simulink model "deltino"  (R2021b)
settings: Solver=VariableStepAuto  StartTime=0.0  StopTime=inf  FixedStep=0.0001  RelTol=1e-3
values from neighbouring files (symbols this model uses):
  alpha1 = 0    [compute_deltino_dyn_parallel.m]
  alpha2 = 2/3*pi    (= 2.09439510239)    [compute_deltino_dyn_parallel.m]
  alpha3 = 4/3*pi    (= 4.18879020479)    [compute_deltino_dyn_parallel.m]
  H = 0.05    [main.m]
  J_T = [J_1', J_2', J_3', J_4']    [main.m]
  K_d = 10    [main.m]
  K_el = 10000    [main.m]
  K_i = 1    [main.m]
  K_p = 200    [main.m]
  K_v = 10    [main.m]
  mu = 0.8    [main.m]
  ni_0 = zeros(18,1)    [main.m]
  offset1 = [l1/2; l2/2; -h/2]    [compute_deltino_dyn_parallel.m]    (also in main.m = [+l1/2; +l2/2; -h/2])
  offset2 = [l1/2; -l2/2; -h/2]    [compute_deltino_dyn_parallel.m]    (also in main.m = [+l1/2; -l2/2; -h/2])
  offset3 = [-l1/2; -l2/2; -h/2]    [compute_deltino_dyn_parallel.m]    (also in main.m)
  offset4 = [-l1/2; l2/2; -h/2]    [compute_deltino_dyn_parallel.m]    (also in main.m = [-l1/2; +l2/2; -h/2])
  p_leg1_0 = forward_kin(theta_leg1_0)    [main.m]
  p_leg2_0 = forward_kin(theta_leg2_0)    [main.m]
  p_leg3_0 = forward_kin(theta_leg3_0)    [main.m]
  p_leg4_0 = forward_kin(theta_leg4_0)    [main.m]
  points_ccw = [+0.1,  0.00 ... (first row only)    [main.m]
  points_cw = [-0.1,  0.00 ... (first row only)    [main.m]
  q_0 = [base_0; ypr_0; theta_leg1_0; ee_leg1_0; theta_leg2_0; ee_leg2_0;        theta_leg3_0; ee_leg3_0; theta_leg4_0; ee_leg4_0;]    [main.m]
  ratio = 2    [main.m]
  steps = 4+2*ratio    (= 8)    [main.m]
  theta_leg1_0 = [pi/6; pi/6; pi/6]    [main.m]
  theta_leg2_0 = [pi/6; pi/6; pi/6]    [main.m]
  theta_leg3_0 = [pi/6; pi/6; pi/6]    [main.m]
  theta_leg4_0 = [pi/6; pi/6; pi/6]    [main.m]
  ts = T/steps    (= 0.1875)    [main.m]
  ts2 = 3*ts    (= 0.5625)    [main.m]
  vel = 0.2    [main.m]
undefined symbols (not defined in the file or in its folder): l1, l_A, l_B, R, radius0, radius1, radius2, theta, WPs
libraries: simulink x14, dspsigops x12
(part 2 of 10)

== matlab function deltino/DELTINO DYNAMICS /compute_S ==
  data: q input; S output
function S  = S(q)
%#codegen

%    This function was generated by the Symbolic Math Toolbox version 9.0.
%    03-May-2022 13:40:15
bx = q(1); by = q(2); bz = q(3);
phi = q(4); zeta = q(5); psi = q(6);
th11 = q(7); th12 = q(8); th13 = q(9);
p1x = q(10); p1y = q(11); p1z = q(12);
th21 = q(13); th22 = q(14); th23 = q(15);
p2x = q(16); p2y = q(17); p2z = q(18);
th31 = q(19); th32 = q(20); th33 = q(21);
p3x = q(22); p3y = q(23); p3z = q(24);
th41 = q(25); th42 = q(26); th43 = q(27);
p4x = q(28); p4y = q(29); p4z = q(30);


t2 = cos(phi);
t3 = cos(psi);
t4 = cos(th11);
t5 = cos(th12);
t6 = cos(th13);
t7 = cos(th21);
t8 = cos(th22);
t9 = cos(th23);
t10 = cos(th31);
t11 = cos(th32);
t12 = cos(th33);
t13 = cos(th41);
t14 = cos(th42);
t15 = cos(th43);
t16 = cos(zeta);
t17 = sin(phi);
t18 = sin(psi);
t19 = sin(th11);
t20 = sin(th12);
t21 = sin(th13);
t22 = sin(th21);
t23 = sin(th22);
t24 = sin(th23);
t25 = sin(th31);
t26 = sin(th32);
t27 = sin(th33);
t28 = sin(th41);
t29 = sin(th42);
t30 = sin(th43);
t31 = sin(zeta);
t32 = -bx;
t33 = -by;
t34 = -bz;
t35 = -p1y;
t36 = -p2y;
t37 = -p3y;
t38 = -p4y;
t39 = -p1z;
t40 = -p2z;
t41 = -p3z;
t42 = -p4z;
t47 = sqrt(3.0);
t43 = t2.*t3;
t44 = t2.*t18;
t45 = t3.*t17;
t46 = t17.*t18;
t48 = t4./5.0;
t49 = t5./5.0;
t50 = t6./5.0;
t51 = t7./5.0;
t52 = t8./5.0;
t53 = t9./5.0;
t54 = t10./5.0;
t55 = t11./5.0;
t56 = t12./5.0;
t57 = t13./5.0;
t58 = t14./5.0;
t59 = t15./5.0;
t60 = t16./2.0;
t61 = t20./5.0;
t62 = t21./5.0;
t63 = t23./5.0;
t64 = t24./5.0;
t65 = t26./5.0;
t66 = t27./5.0;
t67 = t29./5.0;
t68 = t30./5.0;
t69 = t31./2.0;
t73 = t2.*(7.0./2.0e+1);
t74 = t3./1.0e+1;
t75 = t3.*(7.0./2.0e+1);
t76 = t5./1.0e+1;
t77 = t6./1.0e+1;
t78 = t8./1.0e+1;
t79 = t9./1.0e+1;
t80 = t11./1.0e+1;
t81 = t12./1.0e+1;
t82 = t14./1.0e+1;
t83 = t15./1.0e+1;
t84 = t16.*(7.0./2.0e+1);
t85 = t17.*(7.0./2.0e+1);
t86 = t18./1.0e+1;
t87 = t18.*(7.0./2.0e+1);
t88 = t31.*(7.0./2.0e+1);
t91 = (t3.*t19)./5.0;
t92 = (t3.*t22)./5.0;
t93 = (t3.*t25)./5.0;
t94 = (t3.*t28)./5.0;
t97 = (t18.*t19)./5.0;
t98 = (t18.*t22)./5.0;
t99 = (t18.*t25)./5.0;
t100 = (t18.*t28)./5.0;
t103 = (t19.*t31)./5.0;
t104 = (t22.*t31)./5.0;
t105 = (t25.*t31)./5.0;
t106 = (t28.*t31)./5.0;
t131 = (t16.*t17.*t19)./5.0;
t132 = (t16.*t17.*t22)./5.0;
t133 = (t16.*t17.*t25)./5.0;
t134 = (t16.*t17.*t28)./5.0;
t139 = t2.*t16.*(-7.0./2.0e+1);
t140 = t3.*t16.*(-1.0./1.0e+1);
t141 = t3.*t16.*(-7.0./2.0e+1);
t146 = t2.*t31.*(-7.0./2.0e+1);
t147 = t16.*t17.*(-7.0./2.0e+1);
t148 = t16.*t18.*(-1.0./1.0e+1);
t149 = t16.*t18.*(-7.0./2.0e+1);
t151 = t17.*t31.*(-7.0./2.0e+1);
t152 = t18.*t31.*(-7.0./2.0e+1);
t165 = (t2.*t16.*t19)./5.0;
t166 = (t2.*t16.*t22)./5.0;
t167 = (t2.*t16.*t25)./5.0;
t168 = (t2.*t16.*t28)./5.0;
t219 = t3.*t4.*t16.*(-1.0./5.0);
t220 = t3.*t7.*t16.*(-1.0./5.0);
t221 = t3.*t10.*t16.*(-1.0./5.0);
t222 = t3.*t13.*t16.*(-1.0./5.0);
t227 = t3.*t16.*t29.*(-1.0./5.0);
t228 = t3.*t16.*t30.*(-1.0./5.0);
t249 = t16.*t18.*t47.*(-1.0./2.0);
t250 = t18.*t31.*t47.*(-1.0./2.0);
t70 = t31.*t44;
t71 = t31.*t45;
t72 = t31.*t46;
t89 = t31.*t43;
t90 = t2.*t60;
t95 = t2.*t69;
t96 = t17.*t60;
t101 = t17.*t69;
t102 = -t75;
t107 = -t84;
t108 = -t87;
t109 = -t88;
t112 = t43./1.0e+1;
t113 = t43.*(7.0./2.0e+1);
t114 = t16.*t73;
t115 = t16.*t74;
t116 = t16.*t75;
t117 = t44./1.0e+1;
t118 = t45./1.0e+1;
t119 = t44.*(7.0./2.0e+1);
t120 = t45.*(7.0./2.0e+1);
t121 = t31.*t73;
t122 = t17.*t84;
t123 = t31.*t74;
t124 = t16.*t86;
t125 = t18.*t84;
t126 = t46./1.0e+1;
t127 = t46.*(7.0./2.0e+1);
t128 = t31.*t85;
t129 = t31.*t87;
t135 = t31.*t91;
t136 = t31.*t92;
t137 = t31.*t93;
t138 = t31.*t94;
t153 = t3.*t16.*t48;
t154 = t3.*t16.*t49;
t155 = t3.*t16.*t50;
t156 = t3.*t16.*t51;
t157 = t3.*t16.*t52;
t158 = t3.*t16.*t53;
t159 = t3.*t16.*t54;
t160 = t3.*t16.*t55;
t161 = t3.*t16.*t56;
t162 = t3.*t16.*t57;
t163 = t3.*t16.*t58;
t164 = t3.*t16.*t59;
t169 = t16.*t91;
t170 = t3.*t16.*t61;
t171 = t3.*t16.*t62;
t172 = t16.*t92;
t173 = t3.*t16.*t63;
t174 = t3.*t16.*t64;
t175 = t16.*t93;
t176 = t3.*t16.*t65;
t177 = t3.*t16.*t66;
t178 = t16.*t94;
t179 = t3.*t16.*t67;
t180 = t3.*t16.*t68;
t185 = t46.*t84;
t186 = -t131;
t187 = -t132;
t188 = -t133;
t189 = -t134;
t192 = t48+1.0./1.0e+1;
t193 = t49+1.0./1.0e+1;
t194 = t50+1.0./1.0e+1;
t195 = t51+1.0./1.0e+1;
t196 = t52+1.0./1.0e+1;
t197 = t53+1.0./1.0e+1;
t198 = t54-1.0./4.0;
t199 = t54+1.0./1.0e+1;
t200 = t55+1.0./1.0e+1;
t201 = t56+1.0./1.0e+1;
t202 = t80+2.0./5.0;
t203 = t81+2.0./5.0;
t204 = t57-1.0./4.0;
t205 = t57+1.0./1.0e+1;
t206 = t58+1.0./1.0e+1;
t207 = t59+1.0./1.0e+1;
t208 = t82+2.0./5.0;
t209 = t83+2.0./5.0;
t210 = t61+1.0./1.0e+1;
t211 = t62+1.0./1.0e+1;
t212 = t63+1.0./1.0e+1;
t213 = t64+1.0./1.0e+1;
t214 = t65+1.0./1.0e+1;
t215 = t66+1.0./1.0e+1;
t216 = t67+1.0./1.0e+1;
t217 = t68+1.0./1.0e+1;
t225 = t43.*t88;
t226 = t44.*t84;
t233 = t16.*t46.*(-7.0./2.0e+1);
t235 = t48+9.0./2.0e+1;
t236 = t51+9.0./2.0e+1;
t237 = t16.*t43.*(-1.0./1.0e+1);
t238 = t16.*t45.*(-1.0./1.0e+1);
t240 = t16.*t44.*(-7.0./2.0e+1);
t243 = t18.*t47.*t60;
t244 = t18.*t47.*t69;
t245 = t76-3.0./1.0e+1;
t246 = t77-3.0./1.0e+1;
t247 = t78-3.0./1.0e+1;
t248 = t79-3.0./1.0e+1;
t263 = t44.*t47.*t60;
t264 = t46.*t47.*t60;
t271 = t16.*t44.*t47.*(-1.0./2.0);
t272 = t16.*t46.*t47.*(-1.0./2.0);
t368 = t103+t219;
t369 = t104+t220;
t370 = t105+t221;
t371 = t106+t222;
t372 = t60+t250;
t373 = t69+t249;
t404 = t75+t86+t97;
t405 = t75+t86+t100;
t407 = t74+t87+t92;
t408 = t74+t87+t93;
t110 = -t70;
t111 = -t71;
t130 = -t113;
t142 = -t117;
t143 = -t118;
t144 = -t119;
t145 = -t120;
t150 = -t127;
t181 = t70./1.0e+1;
t182 = t71./1.0e+1;
t183 = t70.*(7.0./2.0e+1);
t184 = t71.*(7.0./2.0e+1);
t190 = t72./1.0e+1;
t191 = t72.*(7.0./2.0e+1);
t218 = t16.*t112;
t223 = t89./1.0e+1;
t224 = t16.*t118;
t239 = t89.*(-7.0./2.0e+1);
t241 = t43+t72;
t242 = t46+t89;
t251 = t16.*t198;
t252 = t16.*t204;
t253 = t31.*t192;
t254 = t31.*t195;
t255 = t31.*t198;
t256 = t31.*t199;
t257 = t31.*t202;
t258 = t31.*t203;
t259 = t31.*t204;
t260 = t31.*t205;
t261 = t31.*t208;
t262 = t31.*t209;
t267 = t16.*t235;
t268 = t16.*t236;
t269 = t31.*t235;
t270 = t31.*t236;
t273 = t2.*t16.*t192;
t274 = t2.*t16.*t195;
t275 = t2.*t16.*t199;
t276 = t2.*t16.*t205;
t277 = t16.*t17.*t192;
t278 = t16.*t17.*t195;
t279 = t16.*t17.*t199;
t280 = t16.*t17.*t205;
t281 = t3.*t16.*t210;
t282 = t3.*t16.*t211;
t283 = t3.*t16.*t212;
t284 = t3.*t16.*t213;
t285 = t3.*t16.*t214;
t286 = t3.*t16.*t215;
t287 = t3.*t16.*t216;
t288 = t3.*t16.*t217;
t291 = t31.*t245;
t292 = t31.*t246;
t293 = t31.*t247;
t294 = t31.*t248;
t297 = (t2.*t193)./2.0;
t298 = (t2.*t194)./2.0;
t299 = (t2.*t196)./2.0;
t300 = (t2.*t197)./2.0;
t301 = (t2.*t200)./2.0;
t302 = (t2.*t201)./2.0;
t303 = (t2.*t206)./2.0;
t304 = (t2.*t207)./2.0;
t307 = (t17.*t193)./2.0;
t308 = (t17.*t194)./2.0;
t309 = (t17.*t196)./2.0;
t310 = (t17.*t197)./2.0;
t311 = (t17.*t200)./2.0;
t312 = (t17.*t201)./2.0;
t313 = (t17.*t206)./2.0;
t314 = (t17.*t207)./2.0;
t358 = t60+t244;
t359 = t69+t243;
t360 = (t47.*t193)./2.0;
t361 = (t47.*t194)./2.0;
t362 = (t47.*t196)./2.0;
t363 = (t47.*t197)./2.0;
t364 = (t47.*t200)./2.0;
t365 = (t47.*t201)./2.0;
t366 = (t47.*t206)./2.0;
t367 = (t47.*t207)./2.0;
t409 = t86+t98+t102;
t410 = t86+t99+t102;
t412 = t95+t263;
t413 = t74+t91+t108;
t414 = t74+t94+t108;
t415 = t101+t264;
t429 = t95+t271;
t430 = t101+t272;
t431 = t16.*t407;
t432 = t16.*t408;
t433 = t2.*t404;
t434 = t2.*t405;
t435 = t17.*t404;
t436 = t17.*t405;
t459 = t62.*t373;
t460 = t64.*t373;
t461 = t66.*t373;
t462 = t68.*t373;
t508 = t194.*t373;
t509 = t197.*t373;
t510 = t201.*t373;
t511 = t207.*t373;
t229 = -t181;
t230 = -t182;
t231 = -t183;
t232 = -t184;
t234 = -t191;
t265 = t44+t111;
t266 = t45+t110;
t289 = -t251;
t290 = -t252;
t295 = -t258;
t296 = -t262;
t305 = -t267;
t306 = -t268;
t315 = -t273;
t316 = -t274;
t317 = -t275;
t318 = -t276;
t319 = -t279;
t320 = -t281;
t321 = -t283;
t322 = -t285;
t323 = -t287;
t324 = -t297;
t325 = -t298;
t326 = -t299;
t327 = -t300;
t328 = -t307;
t329 = -t308;
t330 = -t309;
t331 = -t310;
t332 = -t292;
t333 = -t294;
t334 = t48.*t242;
t335 = t49.*t242;
t336 = t50.*t242;
t337 = t51.*t242;
t338 = t52.*t242;
t339 = t53.*t242;
t340 = t54.*t242;
t341 = t55.*t242;
t342 = t56.*t242;
t343 = t57.*t242;
t344 = t58.*t242;
t345 = t59.*t242;
t346 = (t19.*t242)./5.0;
t347 = t61.*t242;
t348 = t62.*t242;
t349 = (t22.*t242)./5.0;
t350 = t63.*t242;
t351 = t64.*t242;
t352 = (t25.*t242)./5.0;
t353 = t65.*t242;
t354 = t66.*t242;
t355 = (t28.*t242)./5.0;
t356 = t67.*t242;
t357 = t68.*t242;
t398 = (t47.*t241)./2.0;
t417 = t73+t301;
t418 = t73+t302;
t419 = t73+t303;
t420 = t73+t304;
t421 = t85+t311;
t422 = t85+t312;
t423 = t85+t313;
t424 = t85+t314;
t425 = t360+7.0./2.0e+1;
t426 = t363+7.0./2.0e+1;
t427 = t365+7.0./2.0e+1;
t428 = t366+7.0./2.0e+1;
t441 = t61.*t359;
t442 = t63.*t359;
t443 = t65.*t359;
t444 = t67.*t359;
t449 = t361-7.0./2.0e+1;
t450 = t362-7.0./2.0e+1;
t451 = t364-7.0./2.0e+1;
t452 = t367-7.0./2.0e+1;
t453 = t16.*t413;
t454 = t16.*t414;
t455 = t2.*t409;
t456 = t2.*t410;
t457 = t17.*t409;
t458 = t17.*t410;
t499 = t193.*t359;
t500 = t196.*t359;
t501 = t200.*t359;
t502 = t206.*t359;
t513 = t241.*t360;
t514 = t241.*t361;
t515 = t241.*t362;
t516 = t241.*t363;
t517 = t241.*t364;
t518 = t241.*t365;
t519 = t241.*t366;
t520 = t241.*t367;
t525 = t47.*t194.*t241.*(-1.0./2.0);
t526 = t47.*t200.*t241.*(-1.0./2.0);
t527 = t47.*t207.*t241.*(-1.0./2.0);
t528 = -t508;
t529 = -t509;
t530 = -t510;
t555 = t155+t459;
t556 = t158+t460;
t557 = t161+t461;
t558 = t164+t462;
t596 = p3z+t34+t255+t432;
t600 = p2z+t34+t270+t431;
t615 = p2z+t34+t88+t115+t125+t172+t254;
t616 = p1z+t34+t88+t115+t149+t169+t253;
t617 = p3z+t34+t109+t115+t125+t175+t256;
t618 = p4z+t34+t109+t115+t149+t178+t260;
t648 = bz+t42+t88+t125+t140+t228+t511;
t374 = t48.*t265;
t375 = t49.*t265;
t376 = t50.*t265;
t377 = t51.*t265;
t378 = t52.*t265;
t379 = t53.*t265;
t380 = t54.*t265;
t381 = t55.*t265;
t382 = t56.*t265;
t383 = t57.*t265;
t384 = t58.*t265;
t385 = t59.*t265;
t386 = (t19.*t265)./5.0;
t387 = t61.*t265;
t388 = t62.*t265;
t389 = (t22.*t265)./5.0;
t390 = t63.*t265;
t391 = t64.*t265;
t392 = (t25.*t265)./5.0;
t393 = t65.*t265;
t394 = t66.*t265;
t395 = (t28.*t265)./5.0;
t396 = t67.*t265;
t397 = t68.*t265;
t399 = t23.*t265.*(-1.0./5.0);
t400 = t24.*t265.*(-1.0./5.0);
t402 = t26.*t265.*(-1.0./5.0);
t403 = t27.*t265.*(-1.0./5.0);
t406 = -t398;
t411 = (t47.*t266)./2.0;
t437 = t73+t324;
t438 = t73+t325;
t439 = t73+t326;
t440 = t73+t327;
t445 = t85+t328;
t446 = t85+t329;
t447 = t85+t330;
t448 = t85+t331;
t463 = t16.*t417;
t464 = t16.*t418;
t465 = t16.*t419;
t466 = t16.*t420;
t467 = t16.*t421;
t468 = t16.*t422;
t469 = t16.*t423;
t470 = t16.*t424;
S = ft_1({bx,by,bz,p1x,p1z,p2x,p2y,p2z,p3x,p3y,p3z,p4x,p4z,t100,t107,t108,t109,t11,t112,t113,t114,t115,t116,t117,t118,t119,t12,t120,t121,t122,t123,t124,t125,t126,t127,t128,t129,t130,t131,t132,t133,t134,t135,t136,t137,t138,t139,t14,t140,t141,t142,t143,t144,t145,t146,t147,t149,t15,t151,t152,t154,t157,t16,t160,t163,t165,t166,t167,t168,t17,t170,t171,t173,t174,t176,t177,t18,t181,t182,t183,t184,t185,t186,t187,t188,t189,t19,t190,t191,t192,t193,t194,t195,t196,t197,t199,t2,t20,t200,t201,t205,t206,t207,t21,t218,t22,t223,t224,t225,t226,t227,t229,t23,t230,t231,t232,t233,t234,t237,t238,t24,t240,t241,t242,t25,t253,t254,t256,t257,t259,t26,t260,t261,t265,t266,t269,t27,t277,t278,t28,t280,t282,t284,t286,t288,t289,t29,t290,t291,t293,t295,t296,t3,t30,t305,t306,t31,t315,t316,t317,t318,t319,t32,t320,t321,t322,t323,t33,t332,t333,t334,t335,t336,t337,t338,t339,t34,t340,t341,t342,t343,t344,t345,t346,t347,t348,t349,t35,t350,t351,t352,t353,t354,t355,t356,t357,t358,t36,t360,t361,t362,t363,t364,t365,t366,t367,t368,t369,t37,t370,t371,t372,t374,t375,t376,t377,t378,t379,t38,t380,t381,t382,t383,t384,t385,t386,t387,t388,t389,t39,t390,t392,t395,t396,t397,t398,t399,t40,t400,t402,t403,t406,t41,t411,t412,t415,t42,t425,t426,t427,t428,t429,t43,t430,t433,t434,t435,t436,t437,t438,t439,t440,t441,t442,t443,t444,t445,t446,t447,t448,t449,t45,t450,t451,t452,t453,t454,t455,t456,t457,t458,t463,t464,t465,t466,t467,t468,t469,t47,t470,t499,t5,t500,t501,t502,t513,t515,t516,t518,t519,t525,t526,t527,t528,t529,t530,t555,t556,t557,t558,t596,t6,t60,t600,t61,t615,t616,t617,t618,t62,t63,t64,t648,t65,t66,t67,t68,t8,t84,t88,t89,t9,t90,t96,t97,t98,t99});
end
function S = ft_1(ct)
bx = ct{1};
by = ct{2};
bz = ct{3};
p1x = ct{4};
p1z = ct{5};
p2x = ct{6};
p2y = ct{7};
p2z = ct{8};
p3x = ct{9};
p3y = ct{10};
p3z = ct{11};
p4x = ct{12};
p4z = ct{13};
t100 = ct{14};
t107 = ct{15};
t108 = ct{16};
t109 = ct{17};
t11 = ct{18};
t112 = ct{19};
t113 = ct{20};
t114 = ct{21};
t115 = ct{22};
t116 = ct{23};
t117 = ct{24};
t118 = ct{25};
t119 = ct{26};
t12 = ct{27};
t120 = ct{28};
t121 = ct{29};
t122 = ct{30};
t123 = ct{31};
t124 = ct{32};
t125 = ct{33};
t126 = ct{34};
t127 = ct{35};
t128 = ct{36};
t129 = ct{37};
t130 = ct{38};
t131 = ct{39};
t132 = ct{40};
t133 = ct{41};
t134 = ct{42};
t135 = ct{43};
t136 = ct{44};
t137 = ct{45};
t138 = ct{46};
t139 = ct{47};
t14 = ct{48};
t140 = ct{49};
t141 = ct{50};
t142 = ct{51};
t143 = ct{52};
t144 = ct{53};
t145 = ct{54};
t146 = ct{55};
t147 = ct{56};
t149 = ct{57};
t15 = ct{58};
t151 = ct{59};
t152 = ct{60};
t154 = ct{61};
t157 = ct{62};
t16 = ct{63};
t160 = ct{64};
t163 = ct{65};
t165 = ct{66};
t166 = ct{67};
t167 = ct{68};
t168 = ct{69};
t17 = ct{70};
t170 = ct{71};
t171 = ct{72};
t173 = ct{73};
t174 = ct{74};
t176 = ct{75};
t177 = ct{76};
t18 = ct{77};
t181 = ct{78};
t182 = ct{79};
t183 = ct{80};
t184 = ct{81};
t185 = ct{82};
t186 = ct{83};
t187 = ct{84};
t188 = ct{85};
t189 = ct{86};
t19 = ct{87};
t190 = ct{88};
t191 = ct{89};
t192 = ct{90};
t193 = ct{91};
t194 = ct{92};
t195 = ct{93};
t196 = ct{94};
t197 = ct{95};
t199 = ct{96};
t2 = ct{97};
t20 = ct{98};
t200 = ct{99};
t201 = ct{100};
t205 = ct{101};
t206 = ct{102};
t207 = ct{103};
t21 = ct{104};
t218 = ct{105};
t22 = ct{106};
t223 = ct{107};
t224 = ct{108};
t225 = ct{109};
t226 = ct{110};
t227 = ct{111};
t229 = ct{112};
t23 = ct{113};
t230 = ct{114};
t231 = ct{115};
t232 = ct{116};
t233 = ct{117};
t234 = ct{118};
t237 = ct{119};
t238 = ct{120};
t24 = ct{121};
t240 = ct{122};
t241 = ct{123};
t242 = ct{124};
t25 = ct{125};
t253 = ct{126};
t254 = ct{127};
t256 = ct{128};
t257 = ct{129};
t259 = ct{130};
t26 = ct{131};
t260 = ct{132};
t261 = ct{133};
t265 = ct{134};
t266 = ct{135};
t269 = ct{136};
t27 = ct{137};
t277 = ct{138};
t278 = ct{139};
t28 = ct{140};
t280 = ct{141};
t282 = ct{142};
t284 = ct{143};
t286 = ct{144};
t288 = ct{145};
t289 = ct{146};
t29 = ct{147};
t290 = ct{148};
t291 = ct{149};
t293 = ct{150};
t295 = ct{151};
t296 = ct{152};
t3 = ct{153};
t30 = ct{154};
t305 = ct{155};
t306 = ct{156};
t31 = ct{157};
t315 = ct{158};
t316 = ct{159};
t317 = ct{160};
t318 = ct{161};
t319 = ct{162};
t32 = ct{163};
t320 = ct{164};
t321 = ct{165};
t322 = ct{166};
t323 = ct{167};
t33 = ct{168};
t332 = ct{169};
t333 = ct{170};
t334 = ct{171};
t335 = ct{172};
t336 = ct{173};
t337 = ct{174};
t338 = ct{175};
t339 = ct{176};
t34 = ct{177};
t340 = ct{178};
t341 = ct{179};
t342 = ct{180};
t343 = ct{181};
t344 = ct{182};
t345 = ct{183};
t346 = ct{184};
t347 = ct{185};
t348 = ct{186};
t349 = ct{187};
t35 = ct{188};
t350 = ct{189};
t351 = ct{190};
t352 = ct{191};
t353 = ct{192};
t354 = ct{193};
t355 = ct{194};
t356 = ct{195};
t357 = ct{196};
t358 = ct{197};
t36 = ct{198};
t360 = ct{199};
t361 = ct{200};
t362 = ct{201};
t363 = ct{202};
t364 = ct{203};
t365 = ct{204};
t366 = ct{205};
t367 = ct{206};
t368 = ct{207};
t369 = ct{208};
t37 = ct{209};
t370 = ct{210};
t371 = ct{211};
t372 = ct{212};
t374 = ct{213};
t375 = ct{214};
t376 = ct{215};
t377 = ct{216};
t378 = ct{217};
t379 = ct{218};
t38 = ct{219};
t380 = ct{220};
t381 = ct{221};
t382 = ct{222};
t383 = ct{223};
t384 = ct{224};
t385 = ct{225};
t386 = ct{226};
t387 = ct{227};
t388 = ct{228};
t389 = ct{229};
t39 = ct{230};
t390 = ct{231};
t392 = ct{232};
t395 = ct{233};
t396 = ct{234};
t397 = ct{235};
t398 = ct{236};
t399 = ct{237};
t40 = ct{238};
t400 = ct{239};
t402 = ct{240};
t403 = ct{241};
t406 = ct{242};
t41 = ct{243};
t411 = ct{244};
t412 = ct{245};
t415 = ct{246};
t42 = ct{247};
t425 = ct{248};
t426 = ct{249};
t427 = ct{250};
t428 = ct{251};
t429 = ct{252};
t43 = ct{253};
t430 = ct{254};
t433 = ct{255};
t434 = ct{256};
t435 = ct{257};
t436 = ct{258};
t437 = ct{259};
t438 = ct{260};
t439 = ct{261};
t440 = ct{262};
t441 = ct{263};
t442 = ct{264};
t443 = ct{265};
t444 = ct{266};
t445 = ct{267};
t446 = ct{268};
t447 = ct{269};
t448 = ct{270};
t449 = ct{271};
t45 = ct{272};
t450 = ct{273};
t451 = ct{274};
t452 = ct{275};
t453 = ct{276};
t454 = ct{277};
t455 = ct{278};
t456 = ct{279};
t457 = ct{280};
t458 = ct{281};
t463 = ct{282};
t464 = ct{283};
t465 = ct{284};
t466 = ct{285};
t467 = ct{286};
t468 = ct{287};
t469 = ct{288};
t47 = ct{289};
t470 = ct{290};
t499 = ct{291};
t5 = ct{292};
t500 = ct{293};
t501 = ct{294};
t502 = ct{295};
t513 = ct{296};
t515 = ct{297};
t516 = ct{298};
t518 = ct{299};
t519 = ct{300};
t525 = ct{301};
t526 = ct{302};
t527 = ct{303};
t528 = ct{304};
t529 = ct{305};
t530 = ct{306};
t555 = ct{307};
t556 = ct{308};
t557 = ct{309};
t558 = ct{310};
t596 = ct{311};
t6 = ct{312};
t60 = ct{313};
t600 = ct{314};
t61 = ct{315};
t615 = ct{316};
t616 = ct{317};
t617 = ct{318};
t618 = ct{319};
t62 = ct{320};
t63 = ct{321};
t64 = ct{322};
t648 = ct{323};
t65 = ct{324};
t66 = ct{325};
t67 = ct{326};
t68 = ct{327};
t8 = ct{328};
t84 = ct{329};
t88 = ct{330};
t89 = ct{331};
t9 = ct{332};
t90 = ct{333};
t96 = ct{334};
t97 = ct{335};
t98 = ct{336};
t99 = ct{337};
t479 = t165+t334;
t480 = t166+t337;
t481 = t167+t340;
t482 = t168+t343;
t485 = t16.*t18.*t425;
t486 = t16.*t18.*t426;
t487 = t16.*t18.*t427;
t488 = t16.*t18.*t428;
t494 = t96+t398;
t495 = t16.*t18.*t449;
t496 = t16.*t18.*t450;
t497 = t16.*t18.*t451;
t498 = t16.*t18.*t452;
t521 = -t499;
t522 = -t500;
t523 = -t501;
t531 = t266.*t360;
t532 = t266.*t361;
t533 = t266.*t362;
t534 = t266.*t363;
t535 = t266.*t364;
t536 = t266.*t365;
t537 = t266.*t366;
t538 = t266.*t367;
t539 = t47.*t194.*t266.*(-1.0./2.0);
t540 = t47.*t197.*t266.*(-1.0./2.0);
t541 = t47.*t201.*t266.*(-1.0./2.0);
t542 = t47.*t207.*t266.*(-1.0./2.0);
t547 = t154+t441;
t548 = t157+t442;
t549 = t160+t443;
t550 = t163+t444;
t583 = t123+t129+t137+t289;
t590 = t123+t129+t136+t306;
t591 = t123+t138+t152+t290;
t599 = t123+t135+t152+t305;
t601 = p4z+t34+t259+t454;
t602 = p1z+t34+t269+t453;
t606 = t2.*(t123+t138+t290+t31.*t108);
t608 = t17.*(t123+t138+t290+t31.*t108);
t609 = t2.*(t123+t135+t305+t31.*t108);
t610 = t17.*(t123+t135+t305+t31.*t108);
t644 = bz+t42+t88+t125+t140+t227+t502;
t646 = p2z+t34+t88+t115+t125+t174+t529;
t649 = t369.*t615;
t650 = p1z+t34+t88+t115+t149+t171+t528;
t651 = p3z+t34+t109+t115+t125+t177+t530;
t652 = t368.*t616;
t653 = t370.*t617;
t655 = t371.*t618;
t666 = p3x+t32+t114+t126+t145+t183+t223+t317+t352;
t667 = p4x+t32+t114+t120+t126+t223+t231+t318+t355;
t669 = p1x+t32+t120+t126+t139+t223+t231+t315+t346;
t670 = p2x+t32+t126+t139+t145+t183+t223+t316+t349;
t680 = t558.*t648;
t401 = -t392;
t416 = -t411;
t471 = t16.*t437;
t472 = t16.*t438;
t473 = t16.*t439;
t474 = t16.*t440;
t475 = t16.*t445;
t476 = t16.*t446;
t477 = t16.*t447;
t478 = t16.*t448;
t483 = -t469;
t484 = -t470;
t503 = t96+t406;
t504 = t186+t374;
t505 = t187+t377;
t506 = t188+t380;
t507 = t189+t383;
t512 = t90+t411;
t543 = t62.*t494;
t544 = t64.*t494;
t545 = t66.*t494;
t546 = t68.*t494;
t575 = t194.*t494;
t576 = t197.*t494;
t577 = t201.*t494;
t578 = t207.*t494;
t603 = t2.*t583;
t604 = t17.*t583;
t605 = t2.*t590;
t607 = t17.*t590;
t613 = -t608;
t614 = -t610;
t635 = p3z+t34+t286+t295+t487;
t636 = bz+t42+t261+t323+t488;
t637 = bz+t41+t257+t322+t497;
t638 = p4z+t34+t288+t296+t498;
t639 = bz+t39+t291+t320+t485;
t640 = p2z+t34+t284+t333+t486;
t641 = p1z+t34+t282+t332+t495;
t642 = bz+t40+t293+t321+t496;
t643 = p2z+t34+t88+t115+t125+t173+t522;
t645 = p1z+t34+t88+t115+t149+t170+t521;
t647 = p3z+t34+t109+t115+t125+t176+t523;
t654 = -t649;
t656 = -t652;
t657 = -t655;
t659 = p4x+t32+t436+t606;
t660 = p1x+t32+t435+t609;
t668 = by+t35+t113+t117+t122+t191+t230+t277+t386;
t671 = by+t38+t113+t117+t147+t191+t230+t280+t395;
t672 = by+t36+t117+t122+t130+t230+t234+t278+t389;
t675 = t550.*t644;
t678 = t556.*t646;
t681 = t555.*t650;
t682 = t557.*t651;
t683 = -t680;
t700 = t481.*t666;
t701 = t482.*t667;
t702 = t479.*t669;
t703 = t480.*t670;
t708 = p3x+t32+t126+t145+t183+t223+t353+t463+t535;
t709 = p4x+t32+t120+t126+t223+t231+t356+t465+t537;
t711 = p3y+t33+t113+t142+t182+t191+t403+t468+t518;
t713 = p3x+t32+t126+t145+t183+t223+t354+t464+t541;
t714 = p4x+t32+t120+t126+t223+t231+t357+t466+t542;
t716 = p3y+t33+t113+t142+t182+t191+t402+t467+t526;
t489 = -t471;
t490 = -t472;
t491 = -t473;
t492 = -t474;
t493 = -t478;
t524 = t90+t416;
t551 = t61.*t503;
t552 = t63.*t503;
t553 = t65.*t503;
t554 = t67.*t503;
t559 = t61.*t512;
t560 = t63.*t512;
t561 = t65.*t512;
t562 = t67.*t512;
t563 = t20.*t512.*(-1.0./5.0);
t565 = t23.*t512.*(-1.0./5.0);
t567 = t26.*t512.*(-1.0./5.0);
t569 = t29.*t512.*(-1.0./5.0);
t579 = t193.*t503;
t580 = t196.*t503;
t581 = t200.*t503;
t582 = t206.*t503;
t584 = t193.*t512;
t585 = t196.*t512;
t586 = t200.*t512;
t587 = t206.*t512;
t588 = -t575;
t589 = -t578;
t611 = -t604;
t612 = -t607;
t619 = t376+t543;
t620 = t379+t544;
t621 = t382+t545;
t622 = t385+t546;
t658 = p3x+t32+t458+t603;
t661 = p2x+t32+t457+t605;
t663 = by+t38+t434+t613;
t664 = by+t35+t433+t614;
t673 = p3y+t33+t113+t122+t142+t182+t191+t319+t401;
t674 = t548.*t643;
t676 = t547.*t645;
t677 = t549.*t647;
t679 = -t675;
t690 = p3y+t33+t113+t122+t142+t182+t191+t403+t577;
t694 = p2y+t33+t113+t142+t147+t182+t191+t400+t576;
t704 = -t700;
t705 = -t668.*(t131-t374);
t706 = -t671.*(t134-t383);
t707 = -t672.*(t132-t377);
t710 = by+t35+t113+t117+t191+t230+t387+t475+t513;
t715 = by+t35+t113+t117+t191+t230+t388+t476+t525;
t717 = by+t38+t113+t117+t191+t230+t396+t483+t519;
t718 = by+t36+t117+t130+t230+t234+t390+t477+t515;
t719 = by+t38+t113+t117+t191+t230+t397+t484+t527;
t749 = -1.0./(t652-t702+t668.*(t131-t374));
t750 = -1.0./(t649-t703+t672.*(t132-t377));
t751 = -1.0./(t655-t701+t671.*(t134-t383));
t757 = t602./(t652-t702+t668.*(t131-t374));
t758 = t600./(t649-t703+t672.*(t132-t377));
t759 = t601./(t655-t701+t671.*(t134-t383));
t764 = (-bx+p1x+t435+t609)./(t652-t702+t668.*(t131-t374));
t765 = (-bx+p4x+t436+t606)./(t655-t701+t671.*(t134-t383));
t564 = t62.*t524;
t566 = t64.*t524;
t568 = t66.*t524;
t570 = t68.*t524;
t571 = t21.*t524.*(-1.0./5.0);
t572 = t24.*t524.*(-1.0./5.0);
t573 = t27.*t524.*(-1.0./5.0);
t574 = t30.*t524.*(-1.0./5.0);
t592 = t194.*t524;
t593 = t197.*t524;
t594 = t201.*t524;
t595 = t207.*t524;
t597 = -t579;
t598 = -t582;
t623 = t335+t563;
t624 = t338+t565;
t625 = t341+t567;
t626 = t344+t569;
t627 = t375+t551;
t628 = t378+t552;
t629 = t381+t553;
t630 = t384+t554;
t662 = by+t37+t456+t611;
t665 = by+t36+t455+t612;
t684 = p3x+t32+t114+t126+t145+t183+t223+t353+t586;
t685 = p4x+t32+t114+t120+t126+t223+t231+t356+t587;
t686 = p1x+t32+t120+t126+t139+t223+t231+t347+t584;
t687 = p2x+t32+t126+t139+t145+t183+t223+t350+t585;
t693 = by+t35+t113+t117+t122+t191+t230+t388+t588;
t695 = p3y+t33+t113+t122+t142+t182+t191+t402+t581;
t697 = p2y+t33+t113+t142+t147+t182+t191+t399+t580;
t698 = by+t38+t113+t117+t147+t191+t230+t397+t589;
t712 = -t673.*(t133-t380);
t720 = p1x+t32+t120+t126+t223+t231+t347+t489+t531;
t721 = p2x+t32+t126+t145+t183+t223+t350+t491+t533;
t722 = p2y+t33+t113+t142+t182+t191+t400+t493+t516;
t723 = p1x+t32+t120+t126+t223+t231+t348+t490+t539;
t724 = p2x+t32+t126+t145+t183+t223+t351+t492+t540;
t727 = t621.*t690;
t731 = t620.*t694;
t745 = t656+t702+t705;
t746 = t654+t703+t707;
t747 = t657+t701+t706;
t752 = -1.0./(-t653+t700+t673.*(t133-t380));
t753 = t602.*t749;
t754 = t600.*t750;
t756 = t601.*t751;
t760 = t749.*(-bx+p1x+t435+t609);
t761 = t751.*(-bx+p4x+t436+t606);
t762 = t661.*t750;
t766 = t664.*t749;
t767 = t663.*t751;
t768 = t661./(t649-t703+t672.*(t132-t377));
t631 = t336+t571;
t632 = t339+t572;
t633 = t342+t573;
t634 = t345+t574;
t688 = p3x+t32+t114+t126+t145+t183+t223+t354+t594;
t689 = p4x+t32+t114+t120+t126+t223+t231+t357+t595;
t691 = p1x+t32+t120+t126+t139+t223+t231+t348+t592;
t692 = p2x+t32+t126+t139+t145+t183+t223+t351+t593;
t696 = by+t35+t113+t117+t122+t191+t230+t387+t597;
t699 = by+t38+t113+t117+t147+t191+t230+t396+t598;
t725 = -t684.*(t561-(t11.*t242)./5.0);
t726 = -t685.*(t562-(t14.*t242)./5.0);
t728 = -t686.*(t559-(t5.*t242)./5.0);
t729 = -t687.*(t560-(t8.*t242)./5.0);
t730 = t619.*t693;
t734 = t629.*t695;
t735 = -t727;
t736 = t622.*t698;
t740 = -t628.*(by+t36+t117+t122+t130+t230+t234+t390-t580);
t741 = -t731;
t744 = t628.*(by+t36+t117+t122+t130+t230+t234+t390-t580);
t748 = t653+t704+t712;
t755 = t596.*t752;
t763 = t658.*t752;
t769 = t665.*t750;
t770 = t662.*t752;
t771 = t662./(-t653+t700+t673.*(t133-t380));
t732 = -t688.*(t568-(t12.*t242)./5.0);
t733 = -t689.*(t570-(t15.*t242)./5.0);
t737 = -t691.*(t564-(t6.*t242)./5.0);
t738 = -t692.*(t566-(t9.*t242)./5.0);
t739 = t627.*t696;
t742 = -t734;
t743 = t630.*t699;
t774 = t674+t729+t744;
t781 = -1.0./(-t677+t734+t684.*(t561-(t11.*t242)./5.0));
t785 = -1.0./(-t682+t727+t688.*(t568-(t12.*t242)./5.0));
t786 = -1.0./(-t678+t731+t692.*(t566-(t9.*t242)./5.0));
t787 = -1.0./(t680-t736+t689.*(t570-(t15.*t242)./5.0));
t793 = t635./(-t682+t727+t688.*(t568-(t12.*t242)./5.0));
t797 = t638./(t680-t736+t689.*(t570-(t15.*t242)./5.0));
t799 = t640./(-t678+t731+t692.*(t566-(t9.*t242)./5.0));
t803 = t708./(-t677+t734+t684.*(t561-(t11.*t242)./5.0));
t814 = t716./(-t677+t734+t684.*(t561-(t11.*t242)./5.0));
t816 = t713./(-t682+t727+t688.*(t568-(t12.*t242)./5.0));
t817 = t711./(-t682+t727+t688.*(t568-(t12.*t242)./5.0));
t820 = t714./(t680-t736+t689.*(t570-(t15.*t242)./5.0));
t825 = t724./(-t678+t731+t692.*(t566-(t9.*t242)./5.0));
t826 = t722./(-t678+t731+t692.*(t566-(t9.*t242)./5.0));
t772 = t676+t728+t739;
t773 = t677+t725+t742;
t775 = t679+t726+t743;
t776 = t681+t730+t737;
t777 = t682+t732+t735;
t778 = t678+t738+t741;
t779 = t683+t733+t736;
t782 = 1.0./t774;
t783 = -1.0./(t675-t743+t685.*(t562-(t14.*t242)./5.0));
t788 = t637.*t781;
t791 = t635.*t785;
t794 = t638.*t787;
t796 = t640.*t786;
t800 = t708.*t781;
t804 = t716.*t781;
t806 = t713.*t785;
t807 = t709./(t675-t743+t685.*(t562-(t14.*t242)./5.0));
t808 = t711.*t785;
t811 = t714.*t787;
t821 = t719.*t787;
t822 = t724.*t786;
t823 = t722.*t786;
t780 = 1.0./t772;
t784 = 1.0./t776;
t789 = t636.*t783;
t792 = t642.*t782;
t801 = t709.*t783;
t809 = t717.*t783;
t810 = t721.*t782;
t813 = t718.*t782;
t790 = t639.*t780;
t795 = t641.*t784;
t802 = t710.*t780;
t805 = t720.*t780;
t812 = t715.*t784;
t818 = t723.*t784;
t819 = -t810;
t798 = -t795;
t815 = -t805;
t824 = -t818;
mt1 = [-1.0,0.0,0.0,0.0,0.0,0.0,t764,t815,t824,0.0,0.0,0.0,t768,t819,t825,0.0,0.0,0.0,t763,t803,t816,0.0,0.0,0.0,t765,t807,t820,0.0,0.0,0.0,0.0,-1.0,0.0,0.0,0.0,0.0,t766,t802,t812,0.0,0.0,0.0,t769,t813,t826,0.0,0.0,0.0,t771,t814,t817,0.0,0.0,0.0,t767,t809,t821,0.0,0.0,0.0,0.0,0.0,-1.0,0.0,0.0,0.0,t757,t790,t798,0.0,0.0,0.0,t758,t792,t799,0.0,0.0,0.0,t755,t788,t793,0.0,0.0,0.0,t759,t789,t797,0.0,0.0,0.0,0.0,0.0,0.0,-1.0,0.0,0.0,t749.*(t669.*(t113+t117+t122+t191+t230+t277+t386)-t668.*(t120+t126+t139+t223+t231+t315+t346)),t780.*(t686.*(t113+t117+t122+t191+t230+t387+t597)-t696.*(t120+t126+t139+t223+t231+t347+t584)),t784.*(t691.*(t113+t117+t122+t191+t230+t388+t588)-t693.*(t120+t126+t139+t223+t231+t348+t592)),0.0,0.0,0.0];
mt2 = [(t672.*(t126+t139+t145+t183+t223+t316+t349)-t670.*(t117+t122+t130+t230+t234+t278+t389))./(t649-t703+t672.*(t132-t377)),-t782.*(t687.*(t113+t142+t182+t191+t399+t580+t17.*t107)+(t126+t139+t145+t183+t223+t350+t585).*(by+t36+t117+t122+t130+t230+t234+t390-t580)),(t692.*(t113+t142+t147+t182+t191+t400+t576)-t694.*(t126+t139+t145+t183+t223+t351+t593))./(-t678+t731+t692.*(t566-(t9.*t242)./5.0)),0.0,0.0,0.0,(t673.*(t114+t126+t145+t183+t223+t317+t352)-t666.*(t113+t122+t142+t182+t191+t319+t401))./(-t653+t700+t673.*(t133-t380))];
mt3 = [(t684.*(t113+t122+t142+t182+t191+t402+t581)-t695.*(t114+t126+t145+t183+t223+t353+t586))./(-t677+t734+t684.*(t561-(t11.*t242)./5.0)),(t688.*(t113+t122+t142+t182+t191+t403+t577)-t690.*(t114+t126+t145+t183+t223+t354+t594))./(-t682+t727+t688.*(t568-(t12.*t242)./5.0)),0.0,0.0,0.0,t751.*(t667.*(t113+t117+t147+t191+t230+t280+t395)-t671.*(t114+t120+t126+t223+t231+t318+t355)),(t699.*(t114+t120+t126+t223+t231+t356+t587)-t685.*(t113+t117+t147+t191+t230+t396+t598))./(t675-t743+t685.*(t562-(t14.*t242)./5.0))];
mt4 = [(t698.*(t114+t120+t126+t223+t231+t357+t595)-t689.*(t113+t117+t147+t191+t230+t397+t589))./(t680-t736+t689.*(t570-(t15.*t242)./5.0)),0.0,0.0,0.0,0.0,0.0,0.0,0.0,-1.0,0.0,t749.*(t616.*(t84+t129-(t3.*t31)./1.0e+1+t16.*t192-(t3.*t19.*t31)./5.0)+t669.*(t121+t218+t240+t2.*t253+(t16.*t19.*t43)./5.0)-t668.*(t128+t224+t233+t17.*t253+(t16.*t19.*t45)./5.0)),-t780.*(t645.*(t107+t123+t152+t193.*t372+t3.*t31.*t61)-t686.*(t121+t218+t240-t193.*t412+t16.*t43.*t61)+t696.*(t128+t224+t233-t193.*t415+t16.*t45.*t61))];
mt5 = [-t784.*(t650.*(t107+t123+t152+t194.*t358+t3.*t31.*t62)-t691.*(t121+t218+t240-t194.*t429+t16.*t43.*t62)+t693.*(t128+t224+t233-t194.*t430+t16.*t45.*t62)),0.0,0.0,0.0,(t615.*(t107+t123+t129+t136-t16.*t195)+t672.*(t128+t185+t224+t17.*t254+(t16.*t22.*t45)./5.0)-t670.*(t121+t218+t226+t2.*t254+(t16.*t22.*t43)./5.0))./(t649-t703+t672.*(t132-t377)),-t782.*(t643.*(t107+t123+t129+t196.*t372+t3.*t31.*t63)-t687.*(t121+t218+t226-t196.*t412+t16.*t43.*t63)+(t128+t185+t224-t196.*t415+t16.*t45.*t63).*(by+t36+t117+t122+t130+t230+t234+t390-t580))];
mt6 = [t786.*(-t646.*(t107+t123+t129+t197.*t358+t3.*t31.*t64)+t694.*(t128+t185+t224-t197.*t430+t16.*t45.*t64)+t692.*(t121+t218+t226-t197.*t429+t16.*t43.*t64)),0.0,0.0,0.0,(-t617.*(t84+t123+t129+t137-t16.*t199)+t673.*(t151+t185+t224+t17.*t256+(t16.*t25.*t45)./5.0)+t666.*(t146+t218+t226+t2.*t256+(t16.*t25.*t43)./5.0))./(-t653+t700+t673.*(t133-t380)),t781.*(-t647.*(t84+t123+t129+t200.*t372+t3.*t31.*t65)+t695.*(t151+t185+t224-t200.*t415+t16.*t45.*t65)+t684.*(t146+t218+t226-t200.*t412+t16.*t43.*t65))];
mt7 = [t785.*(-t651.*(t84+t123+t129+t201.*t358+t3.*t31.*t66)+t690.*(t151+t185+t224-t201.*t430+t16.*t45.*t66)+t688.*(t146+t218+t226-t201.*t429+t16.*t43.*t66)),0.0,0.0,0.0,(t618.*(t84+t123+t138+t152-t16.*t205)-t667.*(t146+t218+t240+t2.*t260+(t16.*t28.*t43)./5.0)+t671.*(t151+t224+t233+t17.*t260+(t16.*t28.*t45)./5.0))./(t655-t701+t671.*(t134-t383)),t783.*(t644.*(t84+t123+t152+t206.*t372+t3.*t31.*t67)+t699.*(t128+t185+t238+t206.*t415-(t16.*t29.*t45)./5.0)-t685.*(t121+t226+t237+t206.*t412-(t16.*t29.*t43)./5.0))];
mt8 = [t787.*(t648.*(t84+t123+t152+t207.*t358+t3.*t31.*t68)+t698.*(t128+t185+t238+t207.*t430-(t16.*t30.*t45)./5.0)-t689.*(t121+t226+t237+t207.*t429-(t16.*t30.*t43)./5.0)),0.0,0.0,0.0,0.0,0.0,0.0,0.0,0.0,-1.0,(-t668.*(t112+t144+t184+t190+(t19.*t241)./5.0)+t669.*(t127+t143+t181+t225-(t19.*t266)./5.0)+t616.*(t116+t124+t16.*t97))./(t652-t702+t668.*(t131-t374)),-t780.*(t645.*(t116+t124+t16.*t18.*t61+t3.*t47.*t60.*t193)-t696.*(t112+t144+t184+t190+t61.*t241-(t47.*t193.*t265)./2.0)+t686.*(t127+t143+t181+t225-(t20.*t266)./5.0+t242.*t360))];
mt9 = [-t784.*(t650.*(t116+t124+t16.*t18.*t62-(t3.*t16.*t47.*t194)./2.0)+t691.*(t89.*(7.0./2.0e+1)+t127+t143+t181-t62.*t266-(t47.*t194.*t242)./2.0)-t693.*(t112+t144+t184+t190+t62.*t241+t265.*t361)),0.0,0.0,0.0,t750.*(t672.*(t112+t119+t190+t232+(t22.*t241)./5.0)+t670.*(t118+t127+t225+t229+(t22.*t266)./5.0)-t615.*(t124+t141+t16.*t98)),t782.*(-t643.*(t124+t141+t16.*t18.*t63+t3.*t47.*t60.*t196)+t687.*(t118+t127+t225+t229+t63.*t266-(t47.*t196.*t242)./2.0)+(t112+t119+t190+t232+t63.*t241-(t47.*t196.*t265)./2.0).*(by+t36+t117+t122+t130+t230+t234+t390-t580))];
mt10 = [t786.*(t646.*(t116-t124-(t16.*t18.*t24)./5.0+t3.*t47.*t60.*t197)-t694.*(t112+t119+t190+t232+t64.*t241+t265.*t363)+t692.*(t118+t127+t225+t229+t64.*t266+t242.*t363)),0.0,0.0,0.0,t752.*(t673.*(t112+t119+t190+t232+(t25.*t241)./5.0)-t666.*(t118+t127+t225+t229+(t25.*t266)./5.0)+t617.*(t124+t141+t16.*t99)),(t647.*(t124+t141+t16.*t18.*t65+t3.*t47.*t60.*t200)+t695.*(t112+t119+t190+t232+t65.*t241-(t47.*t200.*t265)./2.0)-t684.*(t118+t127+t225+t229+t65.*t266-(t47.*t200.*t242)./2.0))./(-t677+t734+t684.*(t561-(t11.*t242)./5.0))];
mt11 = [t785.*(t651.*(t116-t124-(t16.*t18.*t27)./5.0+t3.*t47.*t60.*t201)-t690.*(t112+t119+t190+t232+t66.*t241+t265.*t365)+t688.*(t118+t127+t225+t229+t66.*t266+t242.*t365)),0.0,0.0,0.0,(-t671.*(t112+t144+t184+t190+(t28.*t241)./5.0)+t667.*(t127+t143+t181+t225-(t28.*t266)./5.0)+t618.*(t116+t124+t16.*t100))./(t655-t701+t671.*(t134-t383)),t783.*(t644.*(t116+t124+t16.*t18.*t67+t3.*t47.*t60.*t206)+t699.*(t112+t144+t184+t190+t67.*t241-(t47.*t206.*t265)./2.0)-t685.*(t127+t143+t181+t225-(t29.*t266)./5.0+t242.*t366))];
mt12 = [t787.*(t648.*(t116+t124+t16.*t18.*t68-(t3.*t16.*t47.*t207)./2.0)-t689.*(t89.*(7.0./2.0e+1)+t127+t143+t181-t68.*t266-(t47.*t207.*t242)./2.0)+t698.*(t112+t144+t184+t190+t68.*t241+t265.*t367)),0.0,0.0,0.0,0.0,0.0,0.0,0.0,0.0,0.0,t764,t815,t824,1.0,0.0,0.0,0.0,0.0,0.0,0.0,0.0,0.0,0.0,0.0,0.0,0.0,0.0,0.0,0.0,0.0,0.0,0.0,0.0,0.0,0.0,0.0,0.0,0.0,0.0,0.0,t766,t802,t812,0.0,1.0,0.0,0.0,0.0,0.0,0.0,0.0,0.0,0.0,0.0,0.0,0.0,0.0,0.0,0.0,0.0,0.0,0.0,0.0,0.0,0.0,0.0,0.0,0.0,0.0,0.0,t757,t790,t798,0.0,0.0,1.0,0.0,0.0,0.0,0.0,0.0,0.0,0.0,0.0,0.0,0.0,0.0,0.0,0.0,0.0,0.0,0.0,0.0,0.0,0.0,0.0,0.0,0.0,0.0,0.0,0.0,0.0,0.0,0.0,0.0,0.0,t768,t819,t825,1.0,0.0,0.0,0.0,0.0,0.0,0.0,0.0,0.0,0.0,0.0,0.0,0.0,0.0,0.0,0.0,0.0,0.0,0.0,0.0,0.0,0.0,0.0,0.0,0.0,0.0,0.0,t769,t813,t826,0.0];
mt13 = [1.0,0.0,0.0,0.0,0.0,0.0,0.0,0.0,0.0,0.0,0.0,0.0,0.0,0.0,0.0,0.0,0.0,0.0,0.0,0.0,0.0,0.0,0.0,0.0,0.0,0.0,t758,t792,t799,0.0,0.0,1.0,0.0,0.0,0.0,0.0,0.0,0.0,0.0,0.0,0.0,0.0,0.0,0.0,0.0,0.0,0.0,0.0,0.0,0.0,0.0,0.0,0.0,0.0,0.0,0.0,0.0,0.0,0.0,0.0,0.0,0.0,t763,t803,t816,1.0,0.0,0.0,0.0,0.0,0.0,0.0,0.0,0.0,0.0,0.0,0.0,0.0,0.0,0.0,0.0,0.0,0.0,0.0,0.0,0.0,0.0,0.0,0.0,0.0,0.0,0.0,t771,t814,t817,0.0,1.0,0.0,0.0,0.0,0.0,0.0,0.0,0.0,0.0,0.0,0.0,0.0,0.0,0.0,0.0,0.0,0.0,0.0,0.0,0.0,0.0,0.0,0.0,0.0,0.0,0.0,t755,t788,t793,0.0,0.0,1.0,0.0,0.0,0.0,0.0,0.0,0.0,0.0,0.0,0.0,0.0,0.0,0.0,0.0,0.0,0.0,0.0,0.0,0.0,0.0,0.0,0.0,0.0,0.0,0.0,0.0,0.0,0.0,0.0,0.0,0.0,t765,t807,t820,1.0,0.0,0.0,0.0,0.0,0.0,0.0,0.0,0.0,0.0,0.0,0.0,0.0,0.0,0.0,0.0,0.0,0.0,0.0,0.0,0.0,0.0,0.0,0.0,0.0,0.0,0.0,t767,t809,t821,0.0,1.0,0.0,0.0,0.0,0.0,0.0,0.0,0.0];
mt14 = [0.0,0.0,0.0,0.0,0.0,0.0,0.0,0.0,0.0,0.0,0.0,0.0,0.0,0.0,0.0,0.0,0.0,0.0,t759,t789,t797,0.0,0.0,1.0];
S = reshape([mt1,mt2,mt3,mt4,mt5,mt6,mt7,mt8,mt9,mt10,mt11,mt12,mt13,mt14],30,18);
end
